simulink model "simulation_pid_controller"  (R2019a)
settings: Solver=FixedStepAuto  StartTime=0.0  StopTime=0.5  FixedStep=0.05  RelTol=1e-3
values from neighbouring files (symbols this model uses):
  rho = zeros(10, 1)    [ID_part1.m]
settings Model: Creator=user  LastModifiedBy=user

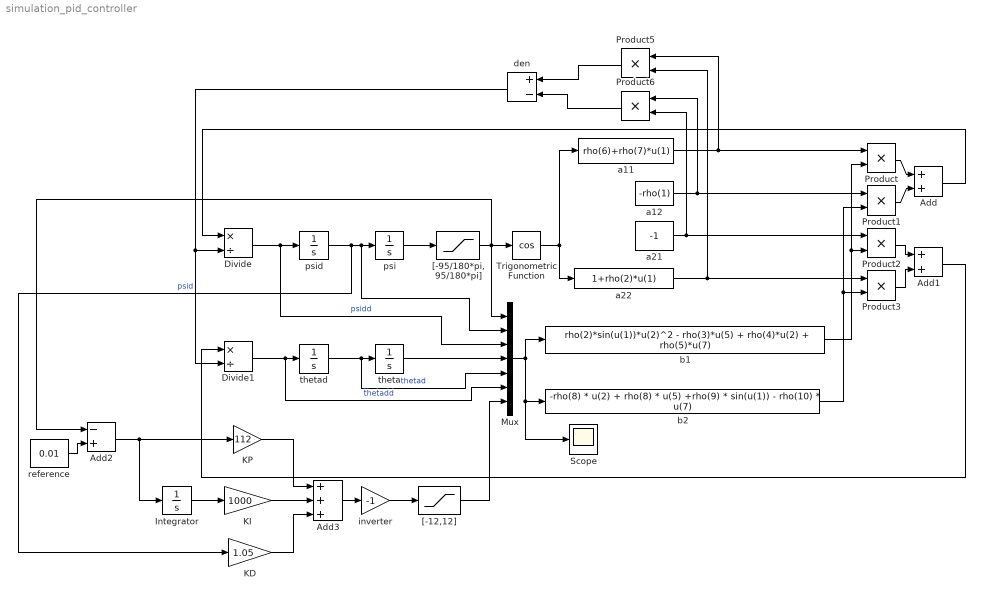
== system simulation_pid_controller ==
  Add : Sum
  Add1 : Sum
  Add2 : Sum  Inputs=-+
  Add3 : Sum  Inputs=+++
  Divide : Product  Inputs=*/
  Divide1 : Product  Inputs=*/
  Integrator : Integrator
  KD : Gain  Gain=1.05
  KI : Gain  Gain=1000
  KP : Gain  Gain=112
  Mux : Mux  Inputs=7
  Product{,1..3,5..6} (6 alike) : Product
  Scope : Scope
  Trigonometric Function : Trigonometry  Operator=cos
  "[-12,12]" : Saturate  UpperLimit=12  LowerLimit=-12
  "[-95/180*pi, 95/180*pi]" : Saturate  UpperLimit=95/180*pi  LowerLimit=-95/180*pi
  a11 : Fcn  Expr=rho(6)+rho(7)*u(1)
  a12 : Constant  Value=-rho(1)
  a21 : Constant  Value=-1
  a22 : Fcn  Expr=1+rho(2)*u(1)
  b1 : Fcn  Expr=rho(2)*sin(u(1))*u(2)^2 - rho(3)*u(5) + rho(4)*u(2) + rho(5)*u(7)
  b2 : Fcn  Expr=-rho(8) * u(2) + rho(8) * u(5) +rho(9) * sin(u(1)) - rho(10) * u(7)
  den : Sum  Inputs=+-
  inverter : Gain  Gain=-1
  psi : Integrator
  psid : Integrator
  reference : Constant  Value=0.01
  theta : Integrator
  thetad : Integrator
  wires:
  psid/1 -> psi/1, Mux/2, KD/1  "psid"
  thetad/1 -> Mux/5, theta/1  "thetad"
  Divide/1 -> Mux/3, psid/1  "psidd"
  Divide1/1 -> Mux/6, thetad/1  "thetadd"
  psi/1 -> "[-95/180*pi, 95/180*pi]"/1
  Mux/1 -> b2/1, Scope/1, b1/1
  "[-95/180*pi, 95/180*pi]"/1 -> Add2/1, Trigonometric Function/1, Mux/1
  Trigonometric Function/1 -> a11/1, a22/1
  a11/1 -> Product5/1, Product/1
  a12/1 -> Product6/1, Product1/1
  b1/1 -> Product2/2, Product/2
  b2/1 -> Product3/2, Product1/2
  a21/1 -> Product6/2, Product2/1
  a22/1 -> Product5/2, Product3/1
  Product/1 -> Add/1
  Product1/1 -> Add/2
  Product2/1 -> Add1/1
  Product3/1 -> Add1/2
  Add/1 -> Divide/1
  Add1/1 -> Divide1/1
  Product5/1 -> den/1
  Product6/1 -> den/2
  den/1 -> Divide/2, Divide1/2
  theta/1 -> Mux/4
  Add2/1 -> KP/1, Integrator/1
  Integrator/1 -> KI/1
  KI/1 -> Add3/2
  KP/1 -> Add3/1
  KD/1 -> Add3/3
  reference/1 -> Add2/2
  Add3/1 -> inverter/1
  inverter/1 -> "[-12,12]"/1
  "[-12,12]"/1 -> Mux/7
